simulink model "engine_throttle"  (Simulink 8.2)
settings: Solver=ode3  StartTime=0  StopTime=1  FixedStep=Ts  RelTol=1e-3
values from neighbouring files (symbols this model uses):
  J = 0.289072836132    [ith_parameter_config.mat]
  K_ITH_POS_OFFSET = 0    [ith_parameter_config.mat]
  K_ITH_POS_PHYS_K = 32.75    [ith_parameter_config.mat]
  K_ITH_POS_PHYS_OFFSET = 574    [ith_parameter_config.mat]
  Kemf = 0.409607180521    [ith_parameter_config.mat]
  Kt = 291.958711155    [ith_parameter_config.mat]
  L = 0.30501560014    [ith_parameter_config.mat]
  R = 30.1778654055    [ith_parameter_config.mat]
  springTorqueCompensation = 0    [ith_parameter_config.mat]
undefined symbols (not defined in the file): angle_init, angle_open, B, Ksp
settings Model: Creator=The MathWorks Inc.  LastModifiedBy=TTI1783  TunableVars=K_ITH_POS_OFFSET,K_ITH_POS_PHYS_K,K_ITH_POS_PHYS_OFFSET,Ksp,angle_init,angle_open,springTorqueCompensation  TunableVarsStorageClass=Auto,Auto,Auto,Auto,Auto,Auto,Auto  TunableVarsTypeQualifier=,,,,,,
settings DataIOCC: ExternalInput=[time3,input3]  LimitDataPoints=off  SaveOutput=off  SaveTime=off
settings OptimizationCC: InlineParams=on  UseFloatMulNetSlope=on  UseSpecifiedMinMax=on  InlineInvariantSignals=on  EnhancedBackFolding=on  ZeroExternalMemoryAtStartup=off  ZeroInternalMemoryAtStartup=off  EfficientFloat2IntCast=on  OptimizeModelRefInitCode=on  LifeSpan=1  BufferReusableBoundary=off
settings DebuggingCC: SaveWithParameterizedLinksMsg=none  MergeDetectMultiDrivingBlocksExec=error  SignalResolutionControl=TryResolveAllWithWarning  SolverPrmCheckMsg=none  MultiTaskDSMMsg=warning  MultiTaskCondExecSysMsg=none  BusObjectLabelMismatch=none
settings HardwareCC: ProdLargestAtomicInteger=Long  ProdLargestAtomicFloat=Double  ProdIntDivRoundTo=Floor  ProdEndianess=LittleEndian  ProdHWDeviceType=ARM Compatible->ARM Cortex
settings RTWCC: SystemTargetFile=ert.tlc  GenCodeOnly=on  GenerateMakefile=off  TemplateMakefile=ert_default_tmf  Description=Embedded Coder  GenerateReport=on  ProcessScript=ert_make_rtw_hook  BuildConfiguration=Faster Runs  IncludeHyperlinkInReport=on  IncludeERTFirstTime=on  GenerateTraceInfo=on  GenerateTraceReport=on  GenerateTraceReportSl=on  GenerateTraceReportSf=on  GenerateTraceReportEml=on  RTWCompilerOptimization=On
settings CodeAppCC: ForceParamTrailComments=on  IgnoreCustomStorageClasses=off  OperatorAnnotations=on  SimulinkDataObjDesc=on  SFDataObjDesc=on  MATLABFcnDesc=on  InsertBlockDesc=on  MATLABSourceComments=on  EnableCustomComments=on  ReqsInCode=on
settings ERTTargetCC: CodeReplacementLibrary=ANSI_C  MultiwordLength=2048  GenerateSampleERTMain=on  IncludeMdlTerminateFcn=off  CombineSignalStateStructs=on  SupportNonFinite=off  SupportContinuousTime=on  ERTCustomFileTemplate=example_file_process.tlc

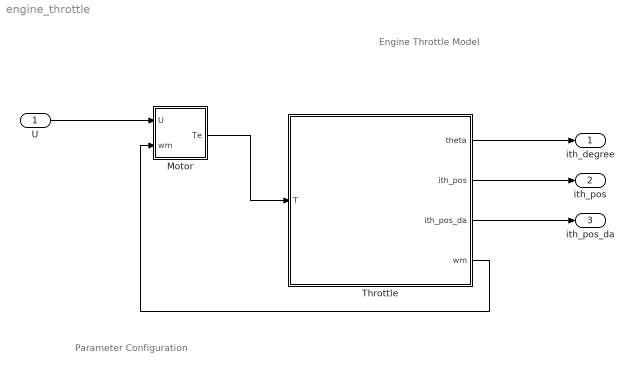
== system engine_throttle ==
  note: Parameter
      | Configuration
  note: Engine Throttle Model
  U : Inport
  Motor : Subsystem
  Throttle : Subsystem  mask{J=J, c=B, k=Ksp, init=angle_init, open_val=angle_open}
      mask prompts: J "Inertia:"; c "Damping:"; k "Stiffness:"; init "Resting Angle:"; open_val "Open Angle:"
      mask init:
      | throttle = imread('spe_engine_throttle.jpg');
      mask Display: image(throttle)
  ith_degree : Outport
  ith_pos : Outport  Port=2
  ith_pos_da : Outport  Port=3
  wires:
  Throttle/1(theta) -> ith_degree/1
  Motor/1(Te) -> Throttle/1(T)
  Throttle/2(ith_pos) -> ith_pos/1
  Throttle/4(wm) -> Motor/2(wm)
  Throttle/3(ith_pos_da) -> ith_pos_da/1
  U/1 -> Motor/1(U)

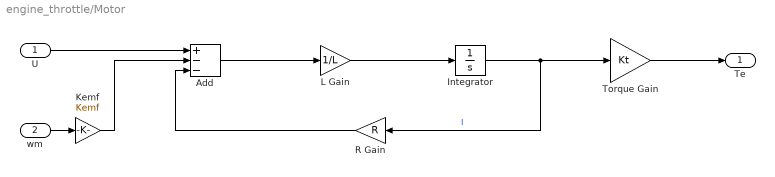
== system engine_throttle/Motor ==
  U : Inport
  wm : Inport  Port=2
  Add : Sum  Inputs=+--
  Integrator : Integrator
  Kemf : Gain  Gain=Kemf
  L Gain : Gain  Gain=1/L
  R Gain : Gain  Gain=R
  Torque Gain : Gain  Gain=Kt  SaturateOnIntegerOverflow=on  OutDataTypeStr=Inherit: Same as input  ParamDataTypeStr=Inherit: Same as input
  Te : Outport
  wires:
  Add/1 -> L Gain/1
  L Gain/1 -> Integrator/1
  wm/1 -> Kemf/1
  Kemf/1 -> Add/2
  R Gain/1 -> Add/3
  Integrator/1 -> Torque Gain/1, R Gain/1  "I"
  Torque Gain/1 -> Te/1
  U/1 -> Add/1

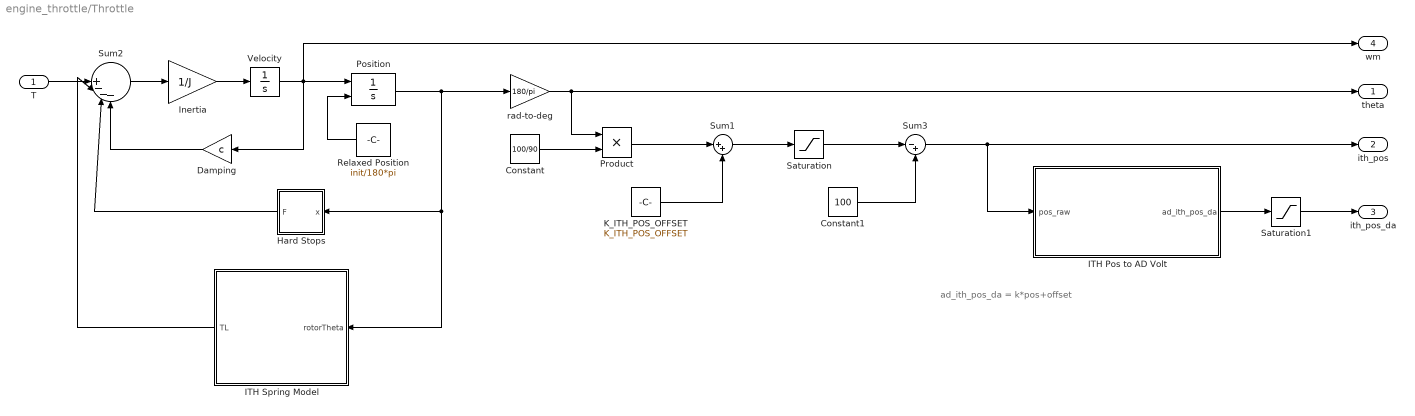
== system engine_throttle/Throttle ==
  note: ad_ith_pos_da = k*pos+offset
  T : Inport
  Constant : Constant  Value=100/90
  Constant1 : Constant  Value=100
  Damping : Gain  Gain=c
  Hard Stops : Subsystem  mask{H=open_val/180*pi, K=2.86e5, L=init/180*pi}
      mask prompts: H "Upper Limit:"; K "Stiffness:"; L "Lower Limit:"
  ITH Pos to AD Volt : Subsystem
  ITH Spring Model : Subsystem  MinMaxOverflowLogging=MinMaxAndOverflow
  Inertia : Gain  Gain=1/J  SaturateOnIntegerOverflow=on  OutDataTypeStr=Inherit: Same as input  ParamDataTypeStr=Inherit: Same as input
  K_ITH_POS_OFFSET : Constant  Value=K_ITH_POS_OFFSET
  Position : Integrator  InitialConditionSource=external
  Product : Product
  Relaxed Position : Constant  Value=init/180*pi
  Saturation : Saturate  UpperLimit=125  LowerLimit=-25
  Saturation1 : Saturate  UpperLimit=4095  LowerLimit=0  OutDataTypeStr=uint16
  Sum1 : Sum  Inputs=|++
  Sum2 : Sum  Inputs=|||+---  SaturateOnIntegerOverflow=on  InputSameDT=on  OutDataTypeStr=Inherit: Same as first input
  Sum3 : Sum  Inputs=|-+
  Velocity : Integrator
  rad-to-deg : Gain  Gain=180/pi
  theta : Outport
  ith_pos : Outport  Port=2
  ith_pos_da : Outport  Port=3
  wm : Outport  Port=4
  wires:
  Damping/1 -> Sum2/4
  Position/1 -> rad-to-deg/1, ITH Spring Model/1(rotorTheta), Hard Stops/1(x)
  Sum2/1 -> Inertia/1
  Inertia/1 -> Velocity/1
  Velocity/1 -> Damping/1, wm/1, Position/1
  T/1 -> Sum2/1
  rad-to-deg/1 -> Product/1, theta/1
  Relaxed Position/1 -> Position/2
  Constant/1 -> Product/2
  ITH Pos to AD Volt/1(ad_ith_pos_da) -> Saturation1/1
  Product/1 -> Sum1/1
  Sum1/1 -> Saturation/1
  K_ITH_POS_OFFSET/1 -> Sum1/2
  Saturation1/1 -> ith_pos_da/1
  Hard Stops/1(F) -> Sum2/3
  ITH Spring Model/1(TL) -> Sum2/2
  Constant1/1 -> Sum3/2
  Saturation/1 -> Sum3/1
  Sum3/1 -> ITH Pos to AD Volt/1(pos_raw), ith_pos/1

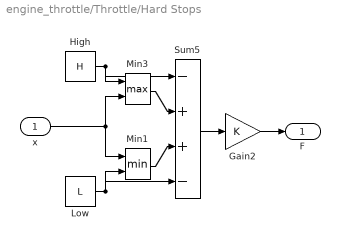
== system engine_throttle/Throttle/Hard Stops ==
  x : Inport
  Gain2 : Gain  Gain=K  SaturateOnIntegerOverflow=on  OutDataTypeStr=Inherit: Same as input  ParamDataTypeStr=Inherit: Same as input
  High : Constant  Value=H
  Low : Constant  Value=L
  Min1 : MinMax  Inputs=2  SaturateOnIntegerOverflow=on  InputSameDT=on
  Min3 : MinMax  Function=max  Inputs=2  SaturateOnIntegerOverflow=on  InputSameDT=on
  Sum5 : Sum  Inputs=-+||+-  SaturateOnIntegerOverflow=on  InputSameDT=on  OutDataTypeStr=Inherit: Same as first input
  F : Outport
  wires:
  Min1/1 -> Sum5/3
  Min3/1 -> Sum5/2
  High/1 -> Min3/1, Sum5/1
  Low/1 -> Sum5/4, Min1/2
  Sum5/1 -> Gain2/1
  x/1 -> Min3/2, Min1/1
  Gain2/1 -> F/1

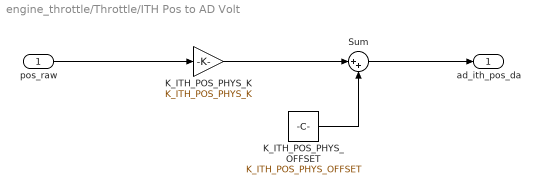
== system engine_throttle/Throttle/ITH Pos to AD Volt ==
  pos_raw : Inport
  K_ITH_POS_PHYS_K : Gain  Gain=K_ITH_POS_PHYS_K
  K_ITH_POS_PHYS_OFFSET : Constant  Value=K_ITH_POS_PHYS_OFFSET
  Sum : Sum  Inputs=|++
  ad_ith_pos_da : Outport
  wires:
  K_ITH_POS_PHYS_K/1 -> Sum/1
  K_ITH_POS_PHYS_OFFSET/1 -> Sum/2
  Sum/1 -> ad_ith_pos_da/1
  pos_raw/1 -> K_ITH_POS_PHYS_K/1

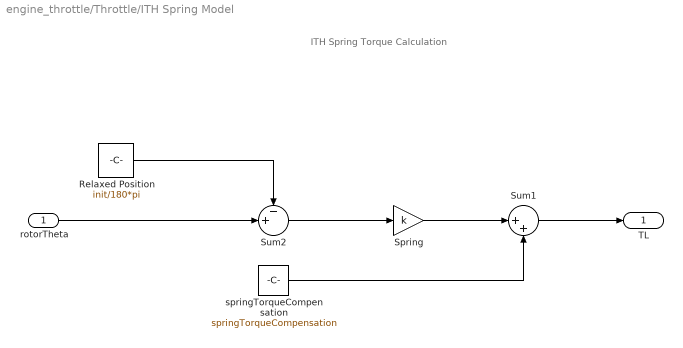
== system engine_throttle/Throttle/ITH Spring Model ==
  note: ITH Spring Torque Calculation
  rotorTheta : Inport
  Relaxed Position : Constant  Value=init/180*pi
  Spring : Gain  Gain=k
  Sum1 : Sum  Inputs=|++
  Sum2 : Sum  Inputs=-+|
  springTorqueCompensation : Constant  Value=springTorqueCompensation
  TL : Outport
  wires:
  Spring/1 -> Sum1/1
  Sum1/1 -> TL/1
  springTorqueCompensation/1 -> Sum1/2
  rotorTheta/1 -> Sum2/2
  Sum2/1 -> Spring/1
  Relaxed Position/1 -> Sum2/1
